simulink model "power_SwitchedReluctanceMotor_v1"  (R2023a)
settings: Solver=FixedStepDiscrete  StartTime=0.0  StopTime=0.5  FixedStep=Ts  RelTol=1e-3  AbsTol=1e-5  EnableMultiTasking=on
PreLoadFcn:
  | Ts=1e-6;
  | 
  | % Magnetisation characteristic table of the switched Reluctance Motor:
  | % Table elements =  Flux linkage, in Wb.
  | 
  | FTBL = [
  |     0             0              0             0             0             0
  |     0.3220    0.3050    0.2280    0.1240    0.0220    0.0170
  |     0.3760    0.3570    0.2770    0.1600    0.0420    0.0340
  |     0.3990    0.3850    0.3000    0.1830    0.0640    0.0500
  |     0.4160    0.4020    0.3200    0.2010    0.0840    0.0670
  |     0.4280    0.4150    0.3340    0.2190    0.1030    0.0840
  |     0.4370    0.4260    0.3480    0.2370    0.1230    0.1010
  |     0.4430    0.4330    0.3590    0.2530    0.1420    0.1170
  |     0.4490    0.4390    0.3710    0.2680    0.1610    0.1340
  |     0.4540    0.4440    0.3820    0.2820    0.1790    0.1510
  |     0.4590    0.4490    0.3920    0.2950    0.1970    0.1680
  |     0.4630    0.4530    0.4020    0.3090    0.2140    0.1840
  |     0.4670    0.4570    0.4110    0.3220    0.2310    0.2010
  |     0.4700    0.4620    0.4190    0.3360    0.2460    0.2180
  |     0.4740    0.4650    0.4270    0.3480    0.2610    0.2350
  |     0.4780    0.4690    0.4330    0.3590    0.2770    0.2510
  |     0.4810    0.4730    0.4380    0.3690    0.2910    0.2680
  |     0.4840    0.4770    0.4440    0.3800    0.3050    0.2850
  |     0.4870    0.4790    0.4480    0.3890    0.3200    0.3020];
  | 
  | % Table columns :  Rotor angles, in degrees.
  | 
  | RotorAngles = [
  |     0             10            20            30            40            45];
  | 
  | % Table rows : Stator current, in A.
  | 
  | StatorCurrents = [ 0:size(FTBL,1)-1] * 25;
  | 
  | % In the Switched Reluctance Motor block, select the "plot magnetization curves"
  | % to plot the corresponding characteristic of the above table.
undefined symbols (not defined in the file): DiscIntNeverNeededParam, find_system
libraries: spsDiodeLib x6, spsIGBTLib x6, spsDCVoltageSourceLib x1, spsSwitchedReluctanceMotorLib x1, spspowerguiLib x1
settings Model: Creator=The MathWorks, Inc.  LastModifiedBy=ravikrishna_g3
settings SolverCC: AutoScaleAbsTol=off  AlgebraicLoopSolver=TrustRegion  InsertRTBMode=Auto
settings DataIOCC: LimitDataPoints=on  SaveFormat=Array  ReturnWorkspaceOutputs=off  SignalLoggingName=sigsOut
settings OptimizationCC: ExpressionDepthLimit=2147483647  InitFltsAndDblsToZero=on  LifeSpan=inf
settings DebuggingCC: UnderspecifiedInitializationDetection=Classic  MergeDetectMultiDrivingBlocksExec=none  CheckExecutionContextPreStartOutputMsg=on  SignalResolutionControl=TryResolveAllWithWarning  MultiTaskDSMMsg=warning  MultiTaskCondExecSysMsg=none  FcnCallInpInsideContextMsg=warning  UnconnectedInputMsg=warning  UnconnectedOutputMsg=warning  UnconnectedLineMsg=warning  StateNameClashWarn=warning  SFUnexpectedBacktrackingDiag=warning  SFNoUnconditionalDefaultTransitionDiag=warning  SFExecutionAtInitializationDiag=none  ArithmeticOperatorsInVariantConditions=warning
settings HardwareCC: ProdBitPerPointer=32  ProdBitPerSizeT=32  ProdBitPerPtrDiffT=32  ProdLargestAtomicFloat=None  ProdIntDivRoundTo=Undefined  ProdEndianess=Unspecified  ProdWordSize=32  ProdHWDeviceType=32-bit Generic  TargetUnknown=on
settings ModelReferenceCC: EnableRefExpFcnMdlSchedulingChecks=on  PropagateSignalLabelsOutOfModel=off
settings SFSimCC: SimUseLocalCustomCode=off  CustomCodeUndefinedFunction=UseInterfaceOnly
settings RTWCC: RTWUseLocalCustomCode=off  DLArmComputeVersion=19.05
settings CodeAppCC: StateflowObjectComments=on
settings GRTTargetCC: TargetLangStandard=C89/C90 (ANSI)  CombineOutputUpdateFcns=off  GRTInterface=on
settings ConfigComp: CovMetricSettings=dw  CovSaveCumulativeToWorkspaceVar=on  CovSaveSingleToWorkspaceVar=on  CovExternalEMLEnable=off  CovSFcnEnable=off
settings SimscapeCC: SimscapeNormalizeSystem=off

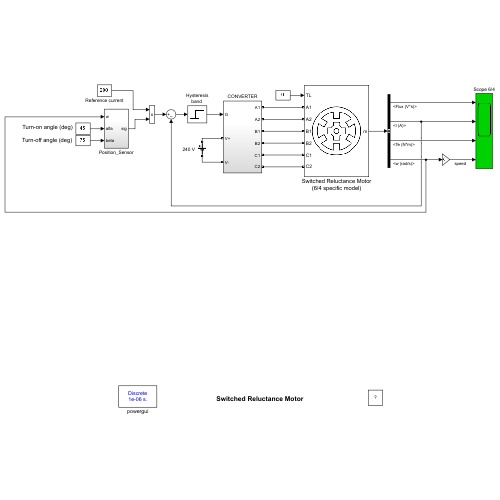
[thumbnail: Simulink's stored preview of the top-level diagram]
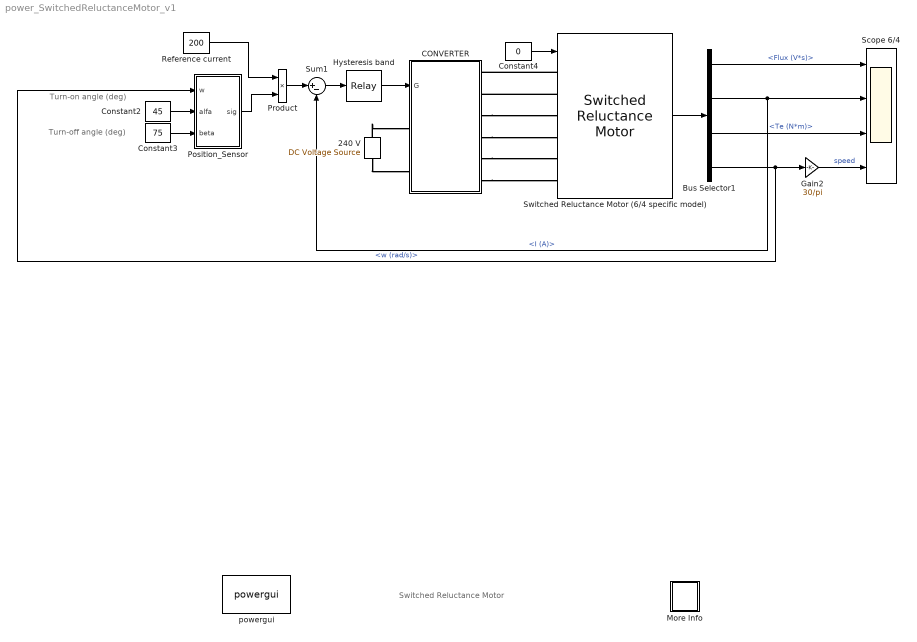
== system power_SwitchedReluctanceMotor_v1 ==
  note: Turn-off angle (deg)
  note: Turn-on angle (deg)
  note: Switched Reluctance Motor
  240 V : spsDCVoltageSourceLib/DC Voltage Source  Amplitude=240  Measurements=None
  Bus Selector1 : BusSelector  OutputSignals=Flux (V*s),I (A),Te (N*m),w (rad/s)
  CONVERTER : Subsystem  LoadFcn=find_system(gcs,'FollowLinks', 'on', 'LookUnderMasks', 'all');
  Constant2 : Constant  Value=45
  Constant3 : Constant  Value=75
  Constant4 : Constant  Value=0
  Gain2 : Gain  Gain=30/pi  SaturateOnIntegerOverflow=on  OutDataTypeStr=Inherit: Same as input  ParamDataTypeStr=Inherit: Same as input
  "Hysteresis band " : Relay  OnSwitchValue=10  OffSwitchValue=-10  SampleTime=Ts
  More Info : Subsystem
      settings: OpenFcn=showdemo(bdroot(gcb))
      mask Display: disp('?')
  Position_Sensor : Subsystem
  Product : Product  SaturateOnIntegerOverflow=on  OutDataTypeStr=Inherit: Same as first input
  Reference current : Constant  Value=200
  Scope 6/4 : Scope  NumInputPorts=4
  Sum1 : Sum  Inputs=|+-  SaturateOnIntegerOverflow=on
  Switched Reluctance Motor (6/4 specific model) : spsSwitchedReluctanceMotorLib/Switched Reluctance Motor  MachineType=6/4  StatorResistance=0.05  Inertia=0.05  Friction=0.02  InitialSpeed=[0,0]  TsPowergui=0  TsBlock=Ts  MachineModel=Specific model  Lq=0.67e-3  Ld=23.6e-3  Lsat=0.15e-3  MaximumCurrent=450  MaximumFluxLinkage=0.486  Source=Dialog  MagnetisationCharacteristic=FTBL  RotorAngleVector=RotorAngles  StatorCurrentVector=StatorCurrents  PlotCurves=off
  powergui : spspowerguiLib/powergui  Priority=2  SimulationMode=Discrete  SampleTime=Ts  frequency=60  Iterations=50  frequencyindice=0  Pbase=100e6  ErrMax=1e-4  UnitsV=kV  UnitsW=MW  buscounter=0  FunctionMessages=off  echomessages=off  EnableUseOfTLC=off  CurrentSourceSwitches=off  DisableSnubberDevices=off  DisableRonSwitches=off  DisableVfSwitches=off  DisplayEquations=off  AutomaticDiscreteSolvers=off  SolverType=Tustin/Backward Euler (TBE)  Interpol=off  ExternalGateDelay=off  methode=off  Ts=0  x0status=blocks  SPID=off  SwTol=0  HookPort=off  NonlinearTolerance=0  nMaxIteration=15  ContinueOnMaxIteration=off  RestoreLinks=warning  ResistiveCurrentMeasurement=off  Frange=[0:2:500]  Ylog=off  Xlog=on  ShowGrid=off  save=off  variable=ZData  structure=0  ZoomFFT=on  StartTime=0.0  cycles=1  DisplayStyle=1  fundamental=60  FreqAxis=off  MaxFrequency=1000  frequencyindicesteady=1  RmsSteady=1  display=off
  wires:
  Constant2/1 -> Position_Sensor/2(alfa)
  Constant3/1 -> Position_Sensor/3(beta)
  Constant4/1 -> Switched Reluctance Motor (6/4 specific model)/1
  Sum1/1 -> "Hysteresis band "/1
  Product/1 -> Sum1/1
  Reference current/1 -> Product/1
  Position_Sensor/1(sig) -> Product/2
  "Hysteresis band "/1 -> CONVERTER/1(G)
  Switched Reluctance Motor (6/4 specific model)/1 -> Bus Selector1/1
  Bus Selector1/1 -> Scope 6/4/1  "<Flux (V*s)>"
  Bus Selector1/2 -> Scope 6/4/2, Sum1/2  "<I (A)>"
  Bus Selector1/3 -> Scope 6/4/3  "<Te (N*m)>"
  Gain2/1 -> Scope 6/4/4  "speed"
  Bus Selector1/4 -> Gain2/1, Position_Sensor/1(w)  "<w (rad/s)>"
  connections:
  240 V/RConn1 -- CONVERTER/LConn1
  240 V/LConn1 -- CONVERTER/LConn2
  Switched Reluctance Motor (6/4 specific model)/LConn1 -- CONVERTER/RConn1
  Switched Reluctance Motor (6/4 specific model)/LConn2 -- CONVERTER/RConn2
  CONVERTER/RConn3 -- Switched Reluctance Motor (6/4 specific model)/LConn3
  CONVERTER/RConn4 -- Switched Reluctance Motor (6/4 specific model)/LConn4
  CONVERTER/RConn5 -- Switched Reluctance Motor (6/4 specific model)/LConn5
  CONVERTER/RConn6 -- Switched Reluctance Motor (6/4 specific model)/LConn6

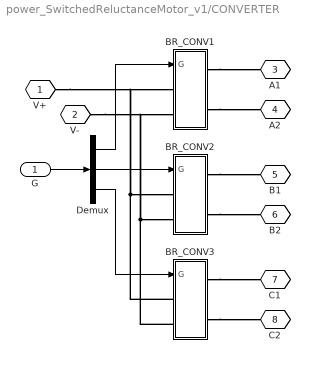
== system power_SwitchedReluctanceMotor_v1/CONVERTER ==
  G : Inport
  BR_CONV1 : Subsystem
  BR_CONV2 : Subsystem
  BR_CONV3 : Subsystem
  Demux : Demux  Outputs=3
      settings: DisplayOption=none
  V+ : PMIOPort  Tag=PMCPort  Side=Left
  V- : PMIOPort  Tag=PMCPort  Port=2  Side=Left
  A1 : PMIOPort  Tag=PMCPort  Port=3  Side=Right
  A2 : PMIOPort  Tag=PMCPort  Port=4  Side=Right
  B1 : PMIOPort  Tag=PMCPort  Port=5  Side=Right
  B2 : PMIOPort  Tag=PMCPort  Port=6  Side=Right
  C1 : PMIOPort  Tag=PMCPort  Port=7  Side=Right
  C2 : PMIOPort  Tag=PMCPort  Port=8  Side=Right
  wires:
  Demux/3 -> BR_CONV3/1(G)
  Demux/1 -> BR_CONV1/1(G)
  Demux/2 -> BR_CONV2/1(G)
  G/1 -> Demux/1
  connections:
  BR_CONV3/RConn2 -- C2/RConn1
  BR_CONV3/RConn1 -- C1/RConn1
  BR_CONV2/RConn2 -- B2/RConn1
  BR_CONV2/RConn1 -- B1/RConn1
  BR_CONV1/RConn2 -- A2/RConn1
  BR_CONV1/RConn1 -- A1/RConn1
  BR_CONV3/LConn2 -- BR_CONV1/LConn2 -- V-/RConn1 -- BR_CONV2/LConn2
  BR_CONV3/LConn1 -- BR_CONV1/LConn1 -- V+/RConn1 -- BR_CONV2/LConn1

== system power_SwitchedReluctanceMotor_v1/More Info ==

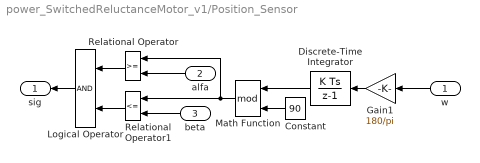
== system power_SwitchedReluctanceMotor_v1/Position_Sensor ==
  w : Inport
  alfa : Inport  Port=2
  beta : Inport  Port=3
  Constant : Constant  Value=90
  Discrete-Time Integrator : DiscreteIntegrator  InitialCondition=[0 -30 -60]  SampleTime=Ts  ICPrevOutput=DiscIntNeverNeededParam  ICPrevScaledInput=DiscIntNeverNeededParam
  Gain1 : Gain  Gain=180/pi  SaturateOnIntegerOverflow=on  OutDataTypeStr=Inherit: Same as input  ParamDataTypeStr=Inherit: Same as input
  Logical Operator : Logic  AllPortsSameDT=off
  Math Function : Math  Operator=mod  SignedPower=on
  Relational Operator : RelationalOperator  InputSameDT=off
  Relational Operator1 : RelationalOperator  Operator=<=  InputSameDT=off
  sig : Outport  VectorParamsAs1DForOutWhenUnconnected=off
  wires:
  Logical Operator/1 -> sig/1
  w/1 -> Gain1/1
  Math Function/1 -> Relational Operator/1, Relational Operator1/1
  Relational Operator1/1 -> Logical Operator/2
  Gain1/1 -> Discrete-Time Integrator/1
  beta/1 -> Relational Operator1/2
  alfa/1 -> Relational Operator/2
  Relational Operator/1 -> Logical Operator/1
  Constant/1 -> Math Function/2
  Discrete-Time Integrator/1 -> Math Function/1

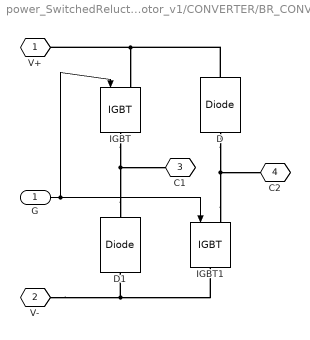
== system power_SwitchedReluctanceMotor_v1/CONVERTER/BR_CONV1 ==
  G : Inport
  D : spsDiodeLib/Diode  Ron=1e-3  Lon=0  Vf=0.8  IC=0  UseSnubber=off  Rs=1000  Cs=inf  Measurements=off
  D1 : spsDiodeLib/Diode  Ron=1e-3  Lon=0  Vf=0.8  IC=0  UseSnubber=off  Rs=1000  Cs=inf  Measurements=off
  IGBT : spsIGBTLib/IGBT  Ron=1e-3  Lon=0  Vf=1  Tf=0  Tt=0  IC=0  Rs=200  Cs=0.1e-6  Measurements=off
  IGBT1 : spsIGBTLib/IGBT  Ron=1e-3  Lon=0  Vf=1  Tf=0  Tt=0  IC=0  Rs=200  Cs=0.1e-6  Measurements=off
  V+ : PMIOPort  Tag=PMCPort  Side=Left
  V- : PMIOPort  Tag=PMCPort  Port=2  Side=Left
  C1 : PMIOPort  Tag=PMCPort  Port=3  Side=Right
  C2 : PMIOPort  Tag=PMCPort  Port=4  Side=Right
  wires:
  G/1 -> IGBT/1, IGBT1/1
  connections:
  D1/LConn1 -- V-/RConn1 -- IGBT1/RConn1
  IGBT1/LConn1 -- D/LConn1 -- C2/RConn1
  D1/RConn1 -- IGBT/RConn1 -- C1/RConn1
  D/RConn1 -- V+/RConn1 -- IGBT/LConn1

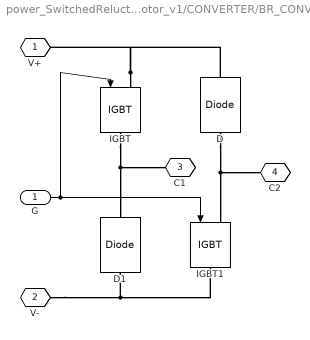
== system power_SwitchedReluctanceMotor_v1/CONVERTER/BR_CONV2 ==
  G : Inport
  D : spsDiodeLib/Diode  Ron=1e-3  Lon=0  Vf=0.8  IC=0  UseSnubber=off  Rs=1000  Cs=inf  Measurements=off
  D1 : spsDiodeLib/Diode  Ron=1e-3  Lon=0  Vf=0.8  IC=0  UseSnubber=off  Rs=1000  Cs=inf  Measurements=off
  IGBT : spsIGBTLib/IGBT  Ron=1e-3  Lon=0  Vf=1  Tf=0  Tt=0  IC=0  Rs=200  Cs=0.1e-6  Measurements=off
  IGBT1 : spsIGBTLib/IGBT  Ron=1e-3  Lon=0  Vf=1  Tf=0  Tt=0  IC=0  Rs=200  Cs=0.1e-6  Measurements=off
  V+ : PMIOPort  Tag=PMCPort  Side=Left
  V- : PMIOPort  Tag=PMCPort  Port=2  Side=Left
  C1 : PMIOPort  Tag=PMCPort  Port=3  Side=Right
  C2 : PMIOPort  Tag=PMCPort  Port=4  Side=Right
  wires:
  G/1 -> IGBT1/1, IGBT/1
  connections:
  IGBT/LConn1 -- V+/RConn1 -- D/RConn1
  IGBT/RConn1 -- D1/RConn1 -- C1/RConn1
  D/LConn1 -- IGBT1/LConn1 -- C2/RConn1
  V-/RConn1 -- D1/LConn1 -- IGBT1/RConn1

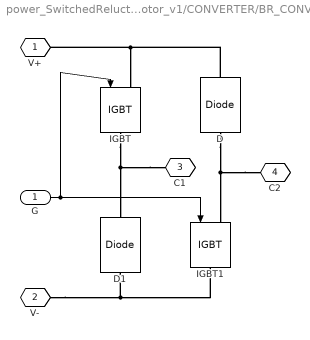
== system power_SwitchedReluctanceMotor_v1/CONVERTER/BR_CONV3 ==
  G : Inport
  D : spsDiodeLib/Diode  Ron=1e-3  Lon=0  Vf=0.8  IC=0  UseSnubber=off  Rs=1000  Cs=inf  Measurements=off
  D1 : spsDiodeLib/Diode  Ron=1e-3  Lon=0  Vf=0.8  IC=0  UseSnubber=off  Rs=1000  Cs=inf  Measurements=off
  IGBT : spsIGBTLib/IGBT  Ron=1e-3  Lon=0  Vf=1  Tf=0  Tt=0  IC=0  Rs=200  Cs=0.1e-6  Measurements=off
  IGBT1 : spsIGBTLib/IGBT  Ron=1e-3  Lon=0  Vf=1  Tf=0  Tt=0  IC=0  Rs=200  Cs=0.1e-6  Measurements=off
  V+ : PMIOPort  Tag=PMCPort  Side=Left
  V- : PMIOPort  Tag=PMCPort  Port=2  Side=Left
  C1 : PMIOPort  Tag=PMCPort  Port=3  Side=Right
  C2 : PMIOPort  Tag=PMCPort  Port=4  Side=Right
  wires:
  G/1 -> IGBT/1, IGBT1/1
  connections:
  IGBT1/RConn1 -- D1/LConn1 -- V-/RConn1
  C2/RConn1 -- IGBT1/LConn1 -- D/LConn1
  C1/RConn1 -- D1/RConn1 -- IGBT/RConn1
  D/RConn1 -- V+/RConn1 -- IGBT/LConn1
